simulink model "foswec"  (R2014a)
settings: Solver=ode45  StartTime=0.0  StopTime=10.0  RelTol=1e-3
undefined symbols (not defined in the file or in its folder): body, constraint, pto
libraries: WECSim_Lib x7
settings Model: Creator=cmichel  LastModifiedBy=cmichel
settings DebuggingCC: MergeDetectMultiDrivingBlocksExec=error

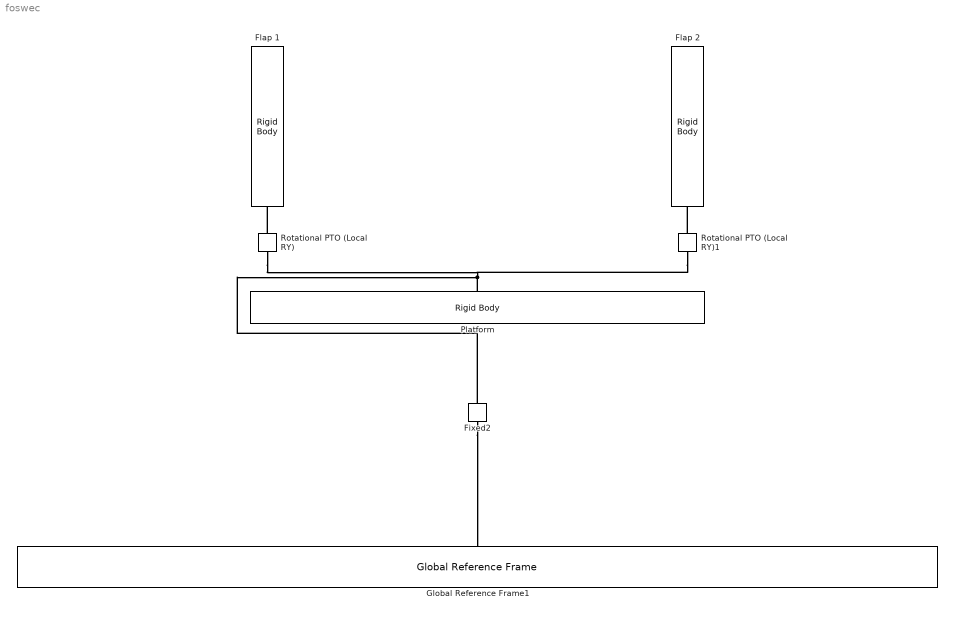
== system foswec ==
  Fixed2 : WECSim_Lib/Constraints/Fixed  constraint=constraint(1)
      settings: AttributesFormatString=%<constraint>
  Flap 1 : WECSim_Lib/Body Elements/Rigid Body  body=body(1)
      settings: AttributesFormatString=%<body>
  Flap 2 : WECSim_Lib/Body Elements/Rigid Body  body=body(2)
      settings: AttributesFormatString=%<body>
  Global Reference Frame1 : WECSim_Lib/Frames/Global Reference Frame  waves=waves  simu=simu
  Platform : WECSim_Lib/Body Elements/Rigid Body  body=body(3)
      settings: AttributesFormatString=%<body>
  Rotational PTO (Local RY) : WECSim_Lib/PTOs/Rotational PTO (Local RY)  pto=pto(1)
      settings: AttributesFormatString=%<pto>
  Rotational PTO (Local RY)1 : WECSim_Lib/PTOs/Rotational PTO (Local RY)  pto=pto(2)
      settings: AttributesFormatString=%<pto>
  connections:
  Rotational PTO (Local RY)1/RConn1 -- Flap 2/RConn1
  Rotational PTO (Local RY)/RConn1 -- Flap 1/RConn1
  Rotational PTO (Local RY)/LConn1 -- Rotational PTO (Local RY)1/LConn1 -- Platform/RConn1 -- Fixed2/RConn1
  Fixed2/LConn1 -- Global Reference Frame1/RConn1

== matlab function foswec/Platform/Wave Radiation Forces Calculation/Convolution-Integral/Fluid Memory ==
  data: check input; v input; F_FM output; ZeroVel input; IRKB input; CTTime input
function F_FM = ConvolutionalIntegral(check,v,ZeroVel,IRKB,CTTime)

%define persistent variables
persistent velocity;
persistent kkk

if check==10
    tmpT = zeros(6,1);
else
    if isempty(velocity)
       velocity = ZeroVel;
       kkk=0;
    else
       kkk=kkk+1;         
       velocity(:,1) = v(:);
       int2=kkk-floor((kkk)/5)*5;
       if int2<0.00000001
          velocity(:,2:end) = velocity(:,1:end-1);
       end
    end 
    
	%integrate
    tmpF = zeros(6,6);
    tmpT = zeros(6,1);
    for kd=1:6
        for kk=1:6
            tmpY=IRKB(:,kd,kk).*velocity(kk,:)';
            tmpF(kd,kk) = trapz(CTTime,tmpY);
        end
        tmpT(kd) = sum(tmpF(kd,1:6));
    end
end
F_FM=tmpT;
end

== matlab function foswec/Platform/Structure/Motion Sensor: Stucture Response/Angle ==
  data: Q input; E output
function E  = EulerAngle(Q)
%#codegen
E=zeros(3,1);
E(1) = atan2( (2*(Q(1)*Q(2)+Q(3)*Q(4))), (1-2* (Q(2)^2+Q(3)^2) ) );
E(2) = asin( 2* (Q(1)*Q(3) - Q(4)*Q(2)));
E(3) = atan2( (2*(Q(1)*Q(4)+Q(2)*Q(3))), (1-2* (Q(3)^2+Q(4)^2) ) );
